simulink model "ILC_pidQuadsim"  (R2024b)
settings: Solver=VariableStepAuto  StartTime=0.0  StopTime=50  RelTol=1e-3
values from neighbouring files (symbols this model uses):
  pwm = (we-4070.3)/0.2685    [mdl_quadrotor.m]
  tsamp_ILC = 0.10    (= 0.1)    [ILC_setup.m]
undefined symbols (not defined in the file or in its folder): A, B, C, D, quad
libraries: slctrlobsolete x4, simulink x3, realtime_pacer_lib x2
(part 2 of 2)

== system ILC_pidQuadsim/Controller2/Attitude_controller/PID_Pitch1 ==
  Setpoint : Inport
  Measured : Inport  Port=2
  1/dt : Gain  Gain=250  OutMin=[-200]  OutMax=[200]
  Kd : Gain  Gain=0  OutMin=[-200]  OutMax=[200]
  Ki : Gain  Gain=0  OutMin=[-200]  OutMax=[200]
  Kp : Gain  Gain=3.5  OutMin=[-200]  OutMax=[200]
  Memory : Memory
  Memory1 : Memory
  Saturation : Saturate  UpperLimit=20  LowerLimit=-20
  Sum1 : Sum  Inputs=|++
  Sum2 : Sum  Inputs=|+-
  Sum5 : Sum  Inputs=+++
  Sum6 : Sum  Inputs=+-|
  dt : Gain  Gain=1/250  OutMin=[-200]  OutMax=[200]
  Adjust : Outport
  wires:
  Measured/1 -> Sum6/2  "measured"
  Setpoint/1 -> Sum6/1  "pid_desired"
  Memory/1 -> Sum2/2  "pid_prevError"
  Ki/1 -> Sum5/2
  Sum5/1 -> Adjust/1
  Kp/1 -> Sum5/1
  Kd/1 -> Sum5/3
  dt/1 -> Sum1/1
  Sum2/1 -> 1/dt/1
  1/dt/1 -> Kd/1
  Sum6/1 -> Sum2/1, Memory/1, dt/1, Kp/1  "pid_error"
  Sum1/1 -> Memory1/1, Saturation/1  "pid_integ"
  Memory1/1 -> Sum1/2
  Saturation/1 -> Ki/1

== system ILC_pidQuadsim/Controller2/Attitude_controller/PID_Pitch3 ==
  Setpoint : Inport
  Measured : Inport  Port=2
  1/dt : Gain  Gain=250  OutMin=[-200]  OutMax=[200]
  Kd : Gain  Gain=0  OutMin=[-200]  OutMax=[200]
  Ki : Gain  Gain=0  OutMin=[-200]  OutMax=[200]
  Kp : Gain  Gain=3.5  OutMin=[-200]  OutMax=[200]
  Memory : Memory
  Memory1 : Memory
  Saturation : Saturate  UpperLimit=20  LowerLimit=-20
  Sum1 : Sum  Inputs=|++
  Sum2 : Sum  Inputs=|+-
  Sum5 : Sum  Inputs=+++
  Sum6 : Sum  Inputs=+-|
  dt : Gain  Gain=1/250  OutMin=[-200]  OutMax=[200]
  Adjust : Outport
  wires:
  Saturation/1 -> Ki/1
  Memory1/1 -> Sum1/2
  Sum1/1 -> Saturation/1, Memory1/1  "pid_integ"
  Sum6/1 -> Kp/1, dt/1, Memory/1, Sum2/1  "pid_error"
  1/dt/1 -> Kd/1
  Sum2/1 -> 1/dt/1
  dt/1 -> Sum1/1
  Kd/1 -> Sum5/3
  Kp/1 -> Sum5/1
  Sum5/1 -> Adjust/1
  Ki/1 -> Sum5/2
  Memory/1 -> Sum2/2  "pid_prevError"
  Setpoint/1 -> Sum6/1  "pid_desired"
  Measured/1 -> Sum6/2  "measured"

== system ILC_pidQuadsim/Controller2/Attitude_controller/PID_Roll_Rate1 ==
  Setpoint : Inport
  Measured : Inport  Port=2
  Derivative : Derivative
  Integrator Limited : Integrator  LimitOutput=on  UpperSaturationLimit=20  LowerSaturationLimit=-20
  Kd : Gain  Gain=0  OutMin=[-200]  OutMax=[200]
  Ki : Gain  Gain=2  OutMin=[-200]  OutMax=[200]
  Kp : Gain  Gain=3.5  OutMin=[-200]  OutMax=[200]
  Scope : Scope
  Sum5 : Sum  Inputs=+++
  Sum6 : Sum  Inputs=+-|
  Adjust : Outport
  wires:
  Derivative/1 -> Kd/1
  Integrator Limited/1 -> Ki/1, Scope/1
  Sum6/1 -> Kp/1, Integrator Limited/1, Derivative/1  "pid_error"
  Kd/1 -> Sum5/3
  Kp/1 -> Sum5/1
  Sum5/1 -> Adjust/1
  Ki/1 -> Sum5/2
  Setpoint/1 -> Sum6/1  "pid_desired"
  Measured/1 -> Sum6/2  "measured"

== system ILC_pidQuadsim/Controller2/Attitude_controller/PID_Roll_Rate2 ==
  Setpoint : Inport
  Measured : Inport  Port=2
  Derivative : Derivative
  Integrator Limited : Integrator  LimitOutput=on  UpperSaturationLimit=20  LowerSaturationLimit=-20
  Kd : Gain  Gain=0  OutMin=[-200]  OutMax=[200]
  Ki : Gain  Gain=2  OutMin=[-200]  OutMax=[200]
  Kp : Gain  Gain=3.5  OutMin=[-200]  OutMax=[200]
  Scope : Scope
  Sum5 : Sum  Inputs=+++
  Sum6 : Sum  Inputs=+-|
  Adjust : Outport
  wires:
  Measured/1 -> Sum6/2  "measured"
  Setpoint/1 -> Sum6/1  "pid_desired"
  Ki/1 -> Sum5/2
  Sum5/1 -> Adjust/1
  Kp/1 -> Sum5/1
  Kd/1 -> Sum5/3
  Sum6/1 -> Derivative/1, Integrator Limited/1, Kp/1  "pid_error"
  Integrator Limited/1 -> Scope/1, Ki/1
  Derivative/1 -> Kd/1

== system ILC_pidQuadsim/Controller2/Control Mixer/Configuration_+ ==
  Pitch : Inport
  Roll : Inport  Port=2
  Yaw : Inport  Port=3
  Tau : Inport  Port=4
  Sum{1,9..12} (5 alike) : Sum  Inputs=|++  InputSameDT=on  SaturateOnIntegerOverflow=on  OutDataTypeStr=Inherit: Same as first input
  Sum3 : Sum  Inputs=|--  InputSameDT=on  SaturateOnIntegerOverflow=on  OutDataTypeStr=Inherit: Same as first input
  Sum5 : Sum  Inputs=|-+  InputSameDT=on  SaturateOnIntegerOverflow=on  OutDataTypeStr=Inherit: Same as first input
  Sum7 : Sum  Inputs=|+-  InputSameDT=on  SaturateOnIntegerOverflow=on  OutDataTypeStr=Inherit: Same as first input
  W1 : Outport
  W2 : Outport  Port=2
  W3 : Outport  Port=3
  W4 : Outport  Port=4
  wires:
  Sum3/1 -> Sum10/1
  Sum1/1 -> Sum9/1
  Sum10/1 -> W2/1
  Sum7/1 -> Sum12/1
  Sum12/1 -> W4/1
  Sum11/1 -> W3/1
  Roll/1 -> Sum7/1, Sum3/1
  Pitch/1 -> Sum5/1, Sum1/1
  Sum9/1 -> W1/1
  Tau/1 -> Sum9/2, Sum10/2, Sum12/2, Sum11/2
  Yaw/1 -> Sum1/2, Sum3/2, Sum5/2, Sum7/2
  Sum5/1 -> Sum11/1

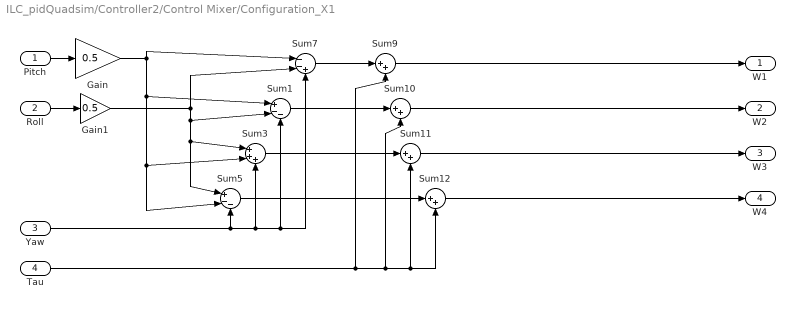
== system ILC_pidQuadsim/Controller2/Control Mixer/Configuration_X1 ==
  Pitch : Inport
  Roll : Inport  Port=2
  Yaw : Inport  Port=3
  Tau : Inport  Port=4
  Gain : Gain  Gain=0.5
  Gain1 : Gain  Gain=0.5
  Sum1 : Sum  Inputs=|+--  InputSameDT=on  SaturateOnIntegerOverflow=on  OutDataTypeStr=Inherit: Same as first input
  Sum{9..12} (4 alike) : Sum  Inputs=|++  InputSameDT=on  SaturateOnIntegerOverflow=on  OutDataTypeStr=Inherit: Same as first input
  Sum3 : Sum  Inputs=|+++  InputSameDT=on  SaturateOnIntegerOverflow=on  OutDataTypeStr=Inherit: Same as first input
  Sum5 : Sum  Inputs=|+--  InputSameDT=on  SaturateOnIntegerOverflow=on  OutDataTypeStr=Inherit: Same as first input
  Sum7 : Sum  Inputs=|--+  InputSameDT=on  SaturateOnIntegerOverflow=on  OutDataTypeStr=Inherit: Same as first input
  W1 : Outport
  W2 : Outport  Port=2
  W3 : Outport  Port=3
  W4 : Outport  Port=4
  wires:
  Sum12/1 -> W4/1
  Sum11/1 -> W3/1
  Sum10/1 -> W2/1
  Sum9/1 -> W1/1
  Gain1/1 -> Sum3/1, Sum5/1, Sum1/2, Sum7/2
  Gain/1 -> Sum3/2, Sum5/2, Sum1/1, Sum7/1
  Pitch/1 -> Gain/1
  Roll/1 -> Gain1/1
  Sum1/1 -> Sum10/1
  Sum7/1 -> Sum9/1
  Sum5/1 -> Sum12/1
  Tau/1 -> Sum9/2, Sum10/2, Sum12/2, Sum11/2
  Yaw/1 -> Sum1/3, Sum7/3, Sum3/3, Sum5/3
  Sum3/1 -> Sum11/1

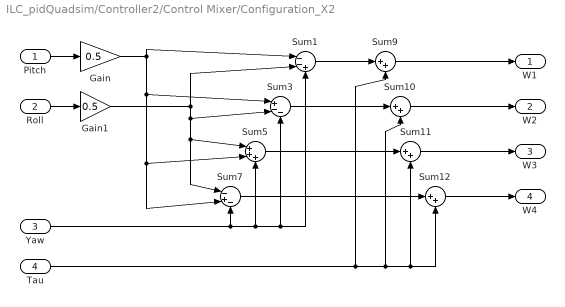
== system ILC_pidQuadsim/Controller2/Control Mixer/Configuration_X2 ==
  Pitch : Inport
  Roll : Inport  Port=2
  Yaw : Inport  Port=3
  Tau : Inport  Port=4
  Gain : Gain  Gain=0.5
  Gain1 : Gain  Gain=0.5
  Sum1 : Sum  Inputs=|--+  InputSameDT=on  SaturateOnIntegerOverflow=on  OutDataTypeStr=Inherit: Same as first input
  Sum{9..12} (4 alike) : Sum  Inputs=|++  InputSameDT=on  SaturateOnIntegerOverflow=on  OutDataTypeStr=Inherit: Same as first input
  Sum3 : Sum  Inputs=|+--  InputSameDT=on  SaturateOnIntegerOverflow=on  OutDataTypeStr=Inherit: Same as first input
  Sum5 : Sum  Inputs=|+++  InputSameDT=on  SaturateOnIntegerOverflow=on  OutDataTypeStr=Inherit: Same as first input
  Sum7 : Sum  Inputs=|-+-  InputSameDT=on  SaturateOnIntegerOverflow=on  OutDataTypeStr=Inherit: Same as first input
  W1 : Outport
  W2 : Outport  Port=2
  W3 : Outport  Port=3
  W4 : Outport  Port=4
  wires:
  Sum5/1 -> Sum11/1
  Yaw/1 -> Sum7/3, Sum5/3, Sum1/3, Sum3/3
  Tau/1 -> Sum11/2, Sum12/2, Sum10/2, Sum9/2
  Sum7/1 -> Sum12/1
  Sum1/1 -> Sum9/1
  Sum3/1 -> Sum10/1
  Roll/1 -> Gain1/1
  Pitch/1 -> Gain/1
  Gain/1 -> Sum3/1, Sum7/2, Sum5/2, Sum1/1
  Gain1/1 -> Sum1/2, Sum3/2, Sum5/1, Sum7/1
  Sum9/1 -> W1/1
  Sum10/1 -> W2/1
  Sum11/1 -> W3/1
  Sum12/1 -> W4/1

== system ILC_pidQuadsim/Controller2/ILC_X/PID ==
  In1 : Inport
  1/Ti : Gain  Gain=1/Ti  SaturateOnIntegerOverflow=on  OutDataTypeStr=Inherit: Same as input  ParamDataTypeStr=Inherit: Same as input
  Integrator : Integrator
  K : Gain  Gain=K  SaturateOnIntegerOverflow=on  OutDataTypeStr=Inherit: Same as input  ParamDataTypeStr=Inherit: Same as input
  Sum1 : Sum  Inputs=+++  InputSameDT=on  SaturateOnIntegerOverflow=on  OutDataTypeStr=Inherit: Same as first input
  Transfer Fcn1 : TransferFcn  Numerator=[Td 0]  Denominator=[Td/10 1]
  Out1 : Outport
  wires:
  In1/1 -> K/1
  K/1 -> 1/Ti/1, Transfer Fcn1/1, Sum1/1
  1/Ti/1 -> Integrator/1
  Sum1/1 -> Out1/1
  Integrator/1 -> Sum1/2
  Transfer Fcn1/1 -> Sum1/3

== system ILC_pidQuadsim/Controller2/ILC_y/PID ==
  In1 : Inport
  1/Ti : Gain  Gain=1/Ti  SaturateOnIntegerOverflow=on  OutDataTypeStr=Inherit: Same as input  ParamDataTypeStr=Inherit: Same as input
  Integrator : Integrator
  K : Gain  Gain=K  SaturateOnIntegerOverflow=on  OutDataTypeStr=Inherit: Same as input  ParamDataTypeStr=Inherit: Same as input
  Sum1 : Sum  Inputs=+++  InputSameDT=on  SaturateOnIntegerOverflow=on  OutDataTypeStr=Inherit: Same as first input
  Transfer Fcn1 : TransferFcn  Numerator=[Td 0]  Denominator=[Td/10 1]
  Out1 : Outport
  wires:
  In1/1 -> K/1
  K/1 -> 1/Ti/1, Transfer Fcn1/1, Sum1/1
  1/Ti/1 -> Integrator/1
  Sum1/1 -> Out1/1
  Integrator/1 -> Sum1/2
  Transfer Fcn1/1 -> Sum1/3

== system ILC_pidQuadsim/Controller2/Position_controller1/PID_Roll_Rate2 ==
  Setpoint : Inport
  Measured : Inport  Port=2
  Derivative : Derivative
  Integrator Limited : Integrator  LimitOutput=on  UpperSaturationLimit=0.1  LowerSaturationLimit=-0.1
  Kd : Gain  Gain=0  OutMin=[-200]  OutMax=[200]
  Ki : Gain  Gain=2  OutMin=[-200]  OutMax=[200]
  Kp : Gain  Gain=30  OutMin=[-200]  OutMax=[200]
  Scope : Scope
  Sum5 : Sum  Inputs=+++
  Sum6 : Sum  Inputs=+-|
  Adjust : Outport
  wires:
  Derivative/1 -> Kd/1
  Integrator Limited/1 -> Ki/1, Scope/1
  Sum6/1 -> Kp/1, Integrator Limited/1, Derivative/1  "pid_error"
  Kd/1 -> Sum5/3
  Kp/1 -> Sum5/1
  Sum5/1 -> Adjust/1
  Ki/1 -> Sum5/2
  Setpoint/1 -> Sum6/1  "pid_desired"
  Measured/1 -> Sum6/2  "measured"

== system ILC_pidQuadsim/Controller2/Position_controller1/PID_Roll_Rate3 ==
  Setpoint : Inport
  Measured : Inport  Port=2
  Derivative : Derivative
  Integrator Limited : Integrator  LimitOutput=on  UpperSaturationLimit=0.1  LowerSaturationLimit=-0.1
  Kd : Gain  Gain=0  OutMin=[-200]  OutMax=[200]
  Ki : Gain  Gain=-2  OutMin=[-200]  OutMax=[200]
  Kp : Gain  Gain=-30  OutMin=[-200]  OutMax=[200]
  Scope : Scope
  Sum5 : Sum  Inputs=+++
  Sum6 : Sum  Inputs=+-|
  Adjust : Outport
  wires:
  Measured/1 -> Sum6/2  "measured"
  Setpoint/1 -> Sum6/1  "pid_desired"
  Ki/1 -> Sum5/2
  Sum5/1 -> Adjust/1
  Kp/1 -> Sum5/1
  Kd/1 -> Sum5/3
  Sum6/1 -> Derivative/1, Integrator Limited/1, Kp/1  "pid_error"
  Integrator Limited/1 -> Scope/1, Ki/1
  Derivative/1 -> Kd/1

== system ILC_pidQuadsim/Controller2/Position_controller1/PID_X2 ==
  Setpoint : Inport
  Measured : Inport  Port=2
  1/dt : Gain  Gain=100  OutMin=[-200]  OutMax=[200]
  Kd : Gain  Gain=0  OutMin=[-200]  OutMax=[200]
  Ki : Gain  OutMin=[-200]  OutMax=[200]
  Kp : Gain  Gain=15  OutMin=[-200]  OutMax=[200]
  Memory : Memory
  Memory1 : Memory
  Saturation : Saturate  UpperLimit=0.1  LowerLimit=-0.1
  Scope1 : Scope
  Scope2 : Scope
  Sum1 : Sum  Inputs=|++
  Sum2 : Sum  Inputs=|+-
  Sum5 : Sum  Inputs=+++
  Sum6 : Sum  Inputs=+-|
  dt : Gain  Gain=1/100  OutMin=[-200]  OutMax=[200]
  Adjust : Outport
  wires:
  Setpoint/1 -> Sum6/1  "pid_desired"
  Memory/1 -> Sum2/2  "pid_prevError"
  Ki/1 -> Sum5/2
  Sum5/1 -> Adjust/1
  Kp/1 -> Sum5/1
  Kd/1 -> Sum5/3
  dt/1 -> Sum1/1
  Sum2/1 -> 1/dt/1
  1/dt/1 -> Kd/1
  Sum6/1 -> Sum2/1, Memory/1, dt/1, Kp/1  "pid_error"
  Sum1/1 -> Memory1/1, Scope1/1, Saturation/1  "pid_integ"
  Memory1/1 -> Sum1/2
  Saturation/1 -> Scope2/1, Ki/1
  Measured/1 -> Sum6/2

== system ILC_pidQuadsim/Controller2/Position_controller1/PID_Y2 ==
  Setpoint : Inport
  Measured : Inport  Port=2
  1/dt : Gain  Gain=100  OutMin=[-200]  OutMax=[200]
  Kd : Gain  Gain=0  OutMin=[-200]  OutMax=[200]
  Ki : Gain  Gain=-1  OutMin=[-200]  OutMax=[200]
  Kp : Gain  Gain=-15  OutMin=[-200]  OutMax=[200]
  Memory : Memory
  Memory1 : Memory
  Saturation : Saturate  UpperLimit=0.1  LowerLimit=-0.1
  Scope1 : Scope
  Scope2 : Scope
  Sum1 : Sum  Inputs=|++
  Sum2 : Sum  Inputs=|+-
  Sum5 : Sum  Inputs=+++
  Sum6 : Sum  Inputs=+-|
  dt : Gain  Gain=1/100  OutMin=[-200]  OutMax=[200]
  Adjust : Outport
  wires:
  Setpoint/1 -> Sum6/1  "pid_desired"
  Memory/1 -> Sum2/2  "pid_prevError"
  Ki/1 -> Sum5/2
  Sum5/1 -> Adjust/1
  Kp/1 -> Sum5/1
  Kd/1 -> Sum5/3
  dt/1 -> Sum1/1
  Sum2/1 -> 1/dt/1
  1/dt/1 -> Kd/1
  Sum6/1 -> Sum2/1, Memory/1, dt/1, Kp/1  "pid_error"
  Sum1/1 -> Memory1/1, Scope1/1, Saturation/1  "pid_integ"
  Memory1/1 -> Sum1/2
  Saturation/1 -> Scope2/1, Ki/1
  Measured/1 -> Sum6/2

== system ILC_pidQuadsim/Controller2/Rate_controller/PID_Pitch_Rate1 ==
  Setpoint : Inport
  Measured : Inport  Port=2
  1/dt : Gain  Gain=500  OutMin=[-200]  OutMax=[200]
  Kd : Gain  Gain=0  OutMin=[-200]  OutMax=[200]
  Ki : Gain  Gain=0  OutMin=[-200]  OutMax=[200]
  Kp : Gain  Gain=70  OutMin=[-200]  OutMax=[200]
  Memory : Memory
  Memory1 : Memory
  Saturation : Saturate  UpperLimit=33  LowerLimit=-33
  Sum1 : Sum  Inputs=|++
  Sum2 : Sum  Inputs=|+-
  Sum5 : Sum  Inputs=+++
  Sum6 : Sum  Inputs=+-|
  dt : Gain  Gain=1/500  OutMin=[-200]  OutMax=[200]
  Adjust : Outport
  wires:
  Measured/1 -> Sum6/2  "measured"
  Setpoint/1 -> Sum6/1  "pid_desired"
  Memory/1 -> Sum2/2  "pid_prevError"
  Ki/1 -> Sum5/2
  Sum5/1 -> Adjust/1
  Kp/1 -> Sum5/1
  Kd/1 -> Sum5/3
  dt/1 -> Sum1/1
  Sum2/1 -> 1/dt/1
  1/dt/1 -> Kd/1
  Sum6/1 -> Sum2/1, Memory/1, dt/1, Kp/1  "pid_error"
  Sum1/1 -> Saturation/1, Memory1/1  "pid_integ"
  Memory1/1 -> Sum1/2
  Saturation/1 -> Ki/1

== system ILC_pidQuadsim/Controller2/Rate_controller/PID_Pitch_Rate3 ==
  Setpoint : Inport
  Measured : Inport  Port=2
  1/dt : Gain  Gain=500  OutMin=[-200]  OutMax=[200]
  Kd : Gain  Gain=0  OutMin=[-200]  OutMax=[200]
  Ki : Gain  Gain=0  OutMin=[-200]  OutMax=[200]
  Kp : Gain  Gain=70  OutMin=[-200]  OutMax=[200]
  Memory : Memory
  Memory1 : Memory
  Saturation : Saturate  UpperLimit=33  LowerLimit=-33
  Sum1 : Sum  Inputs=|++
  Sum2 : Sum  Inputs=|+-
  Sum5 : Sum  Inputs=+++
  Sum6 : Sum  Inputs=+-|
  dt : Gain  Gain=1/500  OutMin=[-200]  OutMax=[200]
  Adjust : Outport
  wires:
  Saturation/1 -> Ki/1
  Memory1/1 -> Sum1/2
  Sum1/1 -> Memory1/1, Saturation/1  "pid_integ"
  Sum6/1 -> Kp/1, dt/1, Memory/1, Sum2/1  "pid_error"
  1/dt/1 -> Kd/1
  Sum2/1 -> 1/dt/1
  dt/1 -> Sum1/1
  Kd/1 -> Sum5/3
  Kp/1 -> Sum5/1
  Sum5/1 -> Adjust/1
  Ki/1 -> Sum5/2
  Memory/1 -> Sum2/2  "pid_prevError"
  Setpoint/1 -> Sum6/1  "pid_desired"
  Measured/1 -> Sum6/2  "measured"

== system ILC_pidQuadsim/Controller2/Rate_controller/PID_Roll_Rate1 ==
  Setpoint : Inport
  Measured : Inport  Port=2
  Derivative : Derivative
  Integrator Limited : Integrator  LimitOutput=on  UpperSaturationLimit=1000  LowerSaturationLimit=-1000
  Kd : Gain  Gain=0  OutMin=[-200]  OutMax=[200]
  Ki : Gain  Gain=0  OutMin=[-200]  OutMax=[200]
  Kp : Gain  Gain=70  OutMin=[-200]  OutMax=[200]
  Scope : Scope
  Sum5 : Sum  Inputs=+++
  Sum6 : Sum  Inputs=+-|
  Adjust : Outport
  wires:
  Derivative/1 -> Kd/1
  Integrator Limited/1 -> Ki/1, Scope/1
  Sum6/1 -> Kp/1, Integrator Limited/1, Derivative/1  "pid_error"
  Kd/1 -> Sum5/3
  Kp/1 -> Sum5/1
  Sum5/1 -> Adjust/1
  Ki/1 -> Sum5/2
  Setpoint/1 -> Sum6/1  "pid_desired"
  Measured/1 -> Sum6/2  "measured"

== system ILC_pidQuadsim/Controller2/Rate_controller/PID_Roll_Rate3 ==
  Setpoint : Inport
  Measured : Inport  Port=2
  Derivative : Derivative
  Integrator Limited : Integrator  LimitOutput=on  UpperSaturationLimit=1000  LowerSaturationLimit=-1000
  Kd : Gain  Gain=0  OutMin=[-200]  OutMax=[200]
  Ki : Gain  Gain=0  OutMin=[-200]  OutMax=[200]
  Kp : Gain  Gain=70  OutMin=[-200]  OutMax=[200]
  Scope : Scope
  Sum5 : Sum  Inputs=+++
  Sum6 : Sum  Inputs=+-|
  Adjust : Outport
  wires:
  Measured/1 -> Sum6/2  "measured"
  Setpoint/1 -> Sum6/1  "pid_desired"
  Ki/1 -> Sum5/2
  Sum5/1 -> Adjust/1
  Kp/1 -> Sum5/1
  Kd/1 -> Sum5/3
  Sum6/1 -> Derivative/1, Integrator Limited/1, Kp/1  "pid_error"
  Integrator Limited/1 -> Scope/1, Ki/1
  Derivative/1 -> Kd/1

== matlab function ILC_pidQuadsim/Quad_Model_X/MATLAB Function ==
  data: uvw input; xyz_dot output; angles input
function xyz_dot  = Position(uvw,angles)
xyz_dot = zeros(3,1);
phi = angles(1); %*pi/180;
theta = angles(2); %*pi/180;
psi = angles(3); %*pi/180;
Tb_o = [cos(theta)*cos(psi)                                cos(theta)*sin(psi)                             -sin(theta)  ;   %BBF > Inertial rotation matrix
        sin(phi)*sin(theta)*cos(psi)-cos(phi)*sin(psi)    sin(phi)*sin(theta)*sin(psi)+cos(phi)*cos(psi)  sin(phi)*cos(theta) ;
        cos(phi)*sin(theta)*cos(psi)+sin(phi)*sin(psi)    cos(phi)*sin(theta)*sin(psi)-sin(phi)*cos(psi)   cos(phi)*cos(theta)];

xyz_dot = (Tb_o')*uvw;
end

== matlab function ILC_pidQuadsim/Quad_Model_X/MATLAB Function1 ==
  data: pqr input; angles_dot output; angles input
function angles_dot  = Angle(pqr,angles)
angles_dot = zeros(3,1);
phi = angles(1); %*pi/180;
theta = angles(2); %*pi/180;

H = [1    sin(phi)*tan(theta)     cos(phi)*tan(theta)
     0       cos(phi)                 -sin(phi)   
     0       sin(phi)/cos(theta)    cos(phi)/cos(theta)];
angles_dot = H*pqr;
end

== matlab function ILC_pidQuadsim/Quad_Model_X/MATLAB Function2 ==
  data: uvw input; uvw_dot output; pqr input; angles input; F input
function uvw_dot  = Forces(uvw,pqr,angles,F)
uvw_dot = zeros(3,1);
Force = [0;0;F];
g_o = [0;0;-9.81];
phi = angles(1); %*pi/180;
theta = angles(2); %*pi/180;
psi = angles(3); %*pi/180;
Tb_o = [cos(theta)*cos(psi)                                cos(theta)*sin(psi)                             -sin(theta)  ;   %BBF > Inertial rotation matrix
        sin(phi)*sin(theta)*cos(psi)-cos(phi)*sin(psi)    sin(phi)*sin(theta)*sin(psi)+cos(phi)*cos(psi)  sin(phi)*cos(theta) ;
        cos(phi)*sin(theta)*cos(psi)+sin(phi)*sin(psi)    cos(phi)*sin(theta)*sin(psi)-sin(phi)*cos(psi)   cos(phi)*cos(theta)];

uvw_dot = Force + Tb_o*g_o - cross(pqr,uvw);

end

== matlab function ILC_pidQuadsim/Quad_Model_X/MATLAB Function3 ==
  data: pqr_dot output; pqr input; M input
function pqr_dot  = Moments(pqr,M)
pqr_dot = zeros(3,1);
Ixx =  1.395e-05;  %2.3951e-5; %1.39e-05; %2.51943e-5; % % %
Iyy = 1.436e-05; %2.3951e-5; %1.436e-05; % 2.54379e-5; % %         %
Izz =  2.173e-05;  %3.2347e-5; %2.173e-05 ; %4.51407e-5; % %         %;%0.160;
J = diag([Ixx Iyy Izz]);    %   I  Flyer rotational inertia matrix     3x3
pqr_dot = inv(J)*(M-cross(pqr,J*pqr));
end
